simulink model "s_heli_2d_ff_lqr_i"  (Simulink 7.0)
settings: Solver=ode1  StartTime=0.0  StopTime=50  FixedStep=0.002  RelTol=1e-3
values from neighbouring files (symbols this model uses):
  g = 9.81    [setup_heli_2d_configuration.m]
  J_eq_p = J_m_p + J_body_p + J_p + J_y    (= 0.0384309870395)    [setup_heli_2d_configuration.m]
  J_eq_y = J_m_y + J_body_y + J_p + J_y + J_shaft    (= 0.0431517259335)    [setup_heli_2d_configuration.m]
  K_pp = K_f_p * r_p    (= 0.20413345)    [setup_heli_2d_configuration.m]
  K_py = K_t_y / R_m_y    (= 0.0068125)    [setup_heli_2d_configuration.m]
  K_yp = K_t_p / R_m_p    (= 0.0219277108434)    [setup_heli_2d_configuration.m]
  K_yy = K_f_y * r_y    (= 0.071988045)    [setup_heli_2d_configuration.m]
  l_cm = ( (m_motor_p + m_shield ) * r_p +  (m_motor_y + m_shield ) * r_y ) / ( m_props )    (= 0.185670125995)    [setup_heli_2d_configuration.m]
  m_heli = 1.3872    [setup_heli_2d_configuration.m]
  SAT_INT_ERR_PITCH = 8    [setup_lab_heli_2d.m]
  SAT_INT_ERR_YAW = 8    [setup_lab_heli_2d.m]
  theta_0 = -40.5*pi/180    (= -0.706858347058)    [setup_lab_heli_2d.m]
  Tr_p = 1    [setup_lab_heli_2d.m]
  Tr_y = 1    [setup_lab_heli_2d.m]
  VMAX_AMP_P = 24    [setup_lab_heli_2d.m]
  VMAX_AMP_Y = 15    [setup_lab_heli_2d.m]
undefined symbols (not defined in the file or in its folder): B_p, B_y, K, Ki
libraries: simulink x4, simulink_extras x4
settings Model: Creator=MLevis  LastModifiedBy=MLevis  ExtModeTrigDuration=5000
settings SolverCC: PositivePriorityOrder=on
settings DebuggingCC: SaveWithParameterizedLinksMsg=none
settings RTWCC: SystemTargetFile=quarc_windows.tlc  TemplateMakefile=quarc_default_tmf  Description=QUARC Win32 Target  ProcessScript=quarc_windows_make_rtw_hook
settings STFCustomTargetCC: TargetFcnLib=ansi_tfl_tmw.mat  TargetPreCompLibLocation=C:\DOCUME~1\ALLUSE~1\APPLIC~1\QUARC\lib\2007b\windows\release  GenFloatMathFcnCalls=ANSI_C  SystemTargetFile=quarc_windows.tlc
settings GRTTargetCC: TargetFcnLib=ansi_tfl_tmw.mat  TargetPreCompLibLocation=C:\DOCUME~1\ALLUSE~1\APPLIC~1\QUARC\lib\2007b\windows\release  CompOptLevelCompliant=off  MatFileLogging=off  ExtMode=on  ExtModeMexFile=quarc_comm

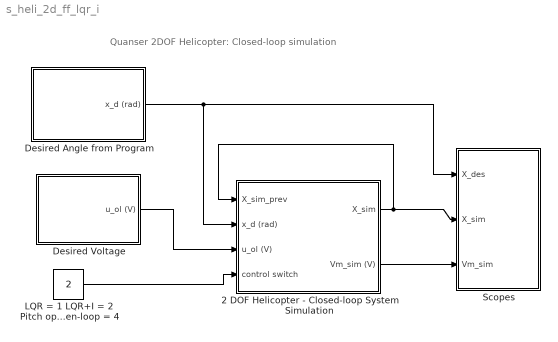
== system s_heli_2d_ff_lqr_i ==
  note: Quanser 2DOF Helicopter: Closed-loop simulation
  2 DOF Helicopter - Closed-loop System Simulation : Subsystem
  Desired Angle from Program : Subsystem
  Desired Voltage : Subsystem
  LQR = 1 LQR+I = 2 Pitch open-loop  = 3 Yaw open-loop = 4 : Constant  Value=2  OutDataType=sfix(16)  OutScaling=2^0
  Scopes : Subsystem
  wires:
  2 DOF Helicopter - Closed-loop System Simulation/1(X_sim) -> 2 DOF Helicopter - Closed-loop System Simulation/1(X_sim_prev), Scopes/2(X_sim)
  2 DOF Helicopter - Closed-loop System Simulation/2(Vm_sim (V)) -> Scopes/3(Vm_sim)
  Desired Angle from Program/1(x_d (rad)) -> Scopes/1(X_des), 2 DOF Helicopter - Closed-loop System Simulation/2(x_d (rad))
  LQR = 1 LQR+I = 2 Pitch open-loop  = 3 Yaw open-loop = 4/1 -> 2 DOF Helicopter - Closed-loop System Simulation/4(control switch)
  Desired Voltage/1(u_ol (V)) -> 2 DOF Helicopter - Closed-loop System Simulation/3(u_ol (V))

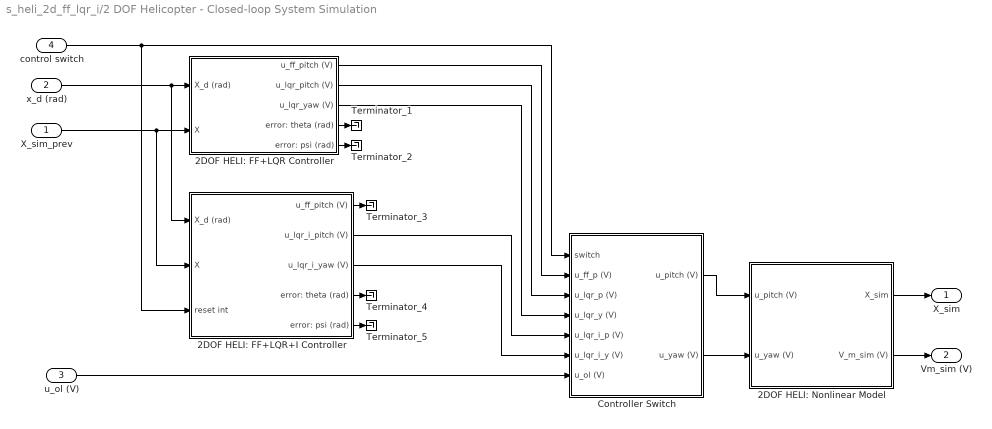
== system s_heli_2d_ff_lqr_i/2 DOF Helicopter - Closed-loop System Simulation ==
  X_sim_prev : Inport  OutDataType=sfix(16)  OutScaling=2^0
  x_d (rad) : Inport  Port=2  OutDataType=sfix(16)  OutScaling=2^0
  u_ol (V) : Inport  Port=3  OutDataType=sfix(16)  OutScaling=2^0
  control switch : Inport  Port=4  OutDataType=sfix(16)  OutScaling=2^0
  2DOF HELI: FF+LQR Controller : Subsystem
  2DOF HELI: FF+LQR+I Controller : Subsystem
  2DOF HELI: Nonlinear Model : Subsystem
  Controller Switch : Subsystem
  Terminator_{1..5} (5 alike) : Terminator
  X_sim : Outport  OutDataType=sfix(16)  OutScaling=2^0
  Vm_sim (V) : Outport  Port=2  OutDataType=sfix(16)  OutScaling=2^0
  wires:
  u_ol (V)/1 -> Controller Switch/7(u_ol (V))
  Controller Switch/2(u_yaw (V)) -> 2DOF HELI: Nonlinear Model/2(u_yaw (V))
  Controller Switch/1(u_pitch (V)) -> 2DOF HELI: Nonlinear Model/1(u_pitch (V))
  x_d (rad)/1 -> 2DOF HELI: FF+LQR+I Controller/1(X_d (rad)), 2DOF HELI: FF+LQR Controller/1(X_d (rad))
  X_sim_prev/1 -> 2DOF HELI: FF+LQR+I Controller/2(X), 2DOF HELI: FF+LQR Controller/2(X)
  2DOF HELI: FF+LQR+I Controller/3(u_lqr_i_yaw (V)) -> Controller Switch/6(u_lqr_i_y (V))
  2DOF HELI: FF+LQR Controller/2(u_lqr_pitch (V)) -> Controller Switch/3(u_lqr_p (V))
  2DOF HELI: FF+LQR Controller/1(u_ff_pitch (V)) -> Controller Switch/2(u_ff_p (V))
  2DOF HELI: FF+LQR Controller/3(u_lqr_yaw (V)) -> Controller Switch/4(u_lqr_y (V))
  2DOF HELI: FF+LQR+I Controller/2(u_lqr_i_pitch (V)) -> Controller Switch/5(u_lqr_i_p (V))
  control switch/1 -> Controller Switch/1(switch), 2DOF HELI: FF+LQR+I Controller/3(reset int)
  2DOF HELI: Nonlinear Model/2(V_m_sim (V)) -> Vm_sim (V)/1
  2DOF HELI: Nonlinear Model/1(X_sim) -> X_sim/1
  2DOF HELI: FF+LQR Controller/4(error: theta (rad)) -> Terminator_1/1
  2DOF HELI: FF+LQR Controller/5(error: psi (rad)) -> Terminator_2/1
  2DOF HELI: FF+LQR+I Controller/1(u_ff_pitch (V)) -> Terminator_3/1
  2DOF HELI: FF+LQR+I Controller/4(error: theta (rad)) -> Terminator_4/1
  2DOF HELI: FF+LQR+I Controller/5(error: psi (rad)) -> Terminator_5/1

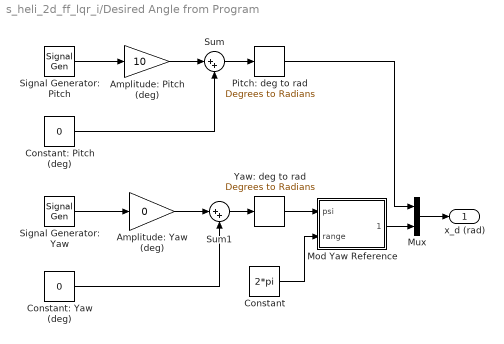
== system s_heli_2d_ff_lqr_i/Desired Angle from Program ==
  Amplitude: Pitch (deg) : Gain  Gain=10  ParameterDataType=sfix(16)  ParameterScaling=2^0  OutDataType=sfix(16)  OutScaling=2^0
  Amplitude: Yaw (deg) : Gain  Gain=0  ParameterDataType=sfix(16)  ParameterScaling=2^0  OutDataType=sfix(16)  OutScaling=2^0
  Constant : Constant  Value=2*pi  OutDataType=sfix(16)  OutScaling=2^0
  Constant: Pitch (deg) : Constant  Value=0  OutDataType=sfix(16)  OutScaling=2^0
  Constant: Yaw (deg) : Constant  Value=0  OutDataType=sfix(16)  OutScaling=2^0
  Mod Yaw Reference : Subsystem
  Mux : Mux  Inputs=2
  Pitch: deg to rad : simulink_extras/Transformations/Degrees to Radians  SystemSampleTime=-1
  Signal Generator: Pitch : SignalGenerator  WaveForm=square  Frequency=0.05
  Signal Generator: Yaw : SignalGenerator  WaveForm=square  Frequency=0.05
  Sum : Sum  Inputs=|++  OutDataType=sfix(16)  OutScaling=2^0
  Sum1 : Sum  Inputs=|++  OutDataType=sfix(16)  OutScaling=2^0
  Yaw: deg to rad : simulink_extras/Transformations/Degrees to Radians  SystemSampleTime=-1
  x_d (rad) : Outport  OutDataType=sfix(16)  OutScaling=2^0
  wires:
  Constant/1 -> Mod Yaw Reference/2(range)
  Yaw: deg to rad/1 -> Mod Yaw Reference/1(psi)
  Mod Yaw Reference/1(mod psi) -> Mux/2
  Pitch: deg to rad/1 -> Mux/1
  Sum/1 -> Pitch: deg to rad/1
  Signal Generator: Pitch/1 -> Amplitude: Pitch (deg)/1
  Amplitude: Pitch (deg)/1 -> Sum/1
  Constant: Pitch (deg)/1 -> Sum/2
  Sum1/1 -> Yaw: deg to rad/1
  Signal Generator: Yaw/1 -> Amplitude: Yaw (deg)/1
  Amplitude: Yaw (deg)/1 -> Sum1/1
  Constant: Yaw (deg)/1 -> Sum1/2
  Mux/1 -> x_d (rad)/1

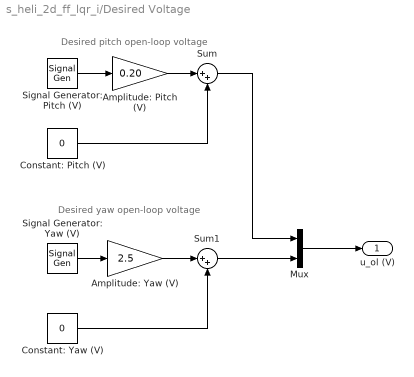
== system s_heli_2d_ff_lqr_i/Desired Voltage ==
  note: Desired pitch open-loop voltage
  note: Desired yaw open-loop voltage
  Amplitude: Pitch (V) : Gain  Gain=0.20  ParameterDataType=sfix(16)  ParameterScaling=2^0  OutDataType=sfix(16)  OutScaling=2^0
  Amplitude: Yaw (V) : Gain  Gain=2.5  ParameterDataType=sfix(16)  ParameterScaling=2^0  OutDataType=sfix(16)  OutScaling=2^0
  Constant: Pitch (V) : Constant  Value=0  OutDataType=sfix(16)  OutScaling=2^0
  Constant: Yaw (V) : Constant  Value=0  OutDataType=sfix(16)  OutScaling=2^0
  Mux : Mux  Inputs=2
  Signal Generator: Pitch (V) : SignalGenerator  WaveForm=square  Frequency=0.5
  Signal Generator: Yaw (V) : SignalGenerator  WaveForm=square  Frequency=0.01
  Sum : Sum  Inputs=|++  OutDataType=sfix(16)  OutScaling=2^0
  Sum1 : Sum  Inputs=|++  OutDataType=sfix(16)  OutScaling=2^0
  u_ol (V) : Outport  OutDataType=sfix(16)  OutScaling=2^0
  wires:
  Constant: Pitch (V)/1 -> Sum/2
  Amplitude: Pitch (V)/1 -> Sum/1
  Signal Generator: Pitch (V)/1 -> Amplitude: Pitch (V)/1
  Constant: Yaw (V)/1 -> Sum1/2
  Amplitude: Yaw (V)/1 -> Sum1/1
  Signal Generator: Yaw (V)/1 -> Amplitude: Yaw (V)/1
  Sum/1 -> Mux/1
  Sum1/1 -> Mux/2
  Mux/1 -> u_ol (V)/1

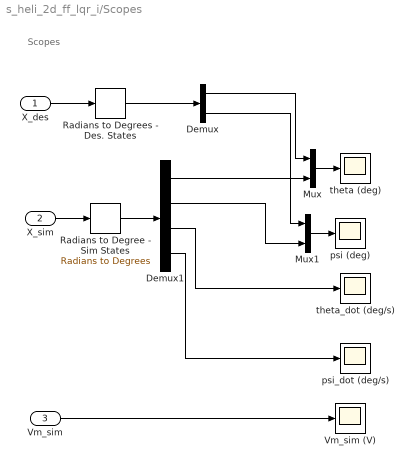
== system s_heli_2d_ff_lqr_i/Scopes ==
  note: Scopes
  X_des : Inport  OutDataType=sfix(16)  OutScaling=2^0
  X_sim : Inport  Port=2  OutDataType=sfix(16)  OutScaling=2^0
  Vm_sim : Inport  Port=3  OutDataType=sfix(16)  OutScaling=2^0
  Demux : Demux  Outputs=2
  Demux1 : Demux
  Mux : Mux  Inputs=2
  Mux1 : Mux  Inputs=2
  Radians to Degree - Sim States : simulink_extras/Transformations/Radians to Degrees  SystemSampleTime=-1
  Radians to Degrees - Des. States : simulink_extras/Transformations/Radians to Degrees  SystemSampleTime=-1
  Vm_sim (V) : Scope
      settings: TickLabels=on  TimeRange=50  YMin=-25  YMax=25  SaveName=ScopeData5  DataFormat=Array
  psi (deg) : Scope
      settings: TickLabels=on  TimeRange=50  YMin=-80  YMax=80  DataFormat=Array
  psi_dot (deg/s) : Scope
      settings: TickLabels=on  TimeRange=50  YMin=-300  YMax=300  SaveName=ScopeData3  DataFormat=Array
  theta (deg) : Scope
      settings: TickLabels=on  TimeRange=50  YMin=-15  YMax=15  DataFormat=Array
  theta_dot (deg/s) : Scope
      settings: TickLabels=on  TimeRange=50  YMin=-300  YMax=300  SaveName=ScopeData2  DataFormat=Array
  wires:
  Vm_sim/1 -> Vm_sim (V)/1
  Radians to Degrees - Des. States/1 -> Demux/1
  Demux1/2 -> Mux1/2
  Demux/2 -> Mux1/1
  Demux1/1 -> Mux/2
  Demux/1 -> Mux/1
  X_des/1 -> Radians to Degrees - Des. States/1
  X_sim/1 -> Radians to Degree - Sim States/1
  Radians to Degree - Sim States/1 -> Demux1/1
  Mux/1 -> theta (deg)/1
  Mux1/1 -> psi (deg)/1
  Demux1/3 -> theta_dot (deg/s)/1
  Demux1/4 -> psi_dot (deg/s)/1

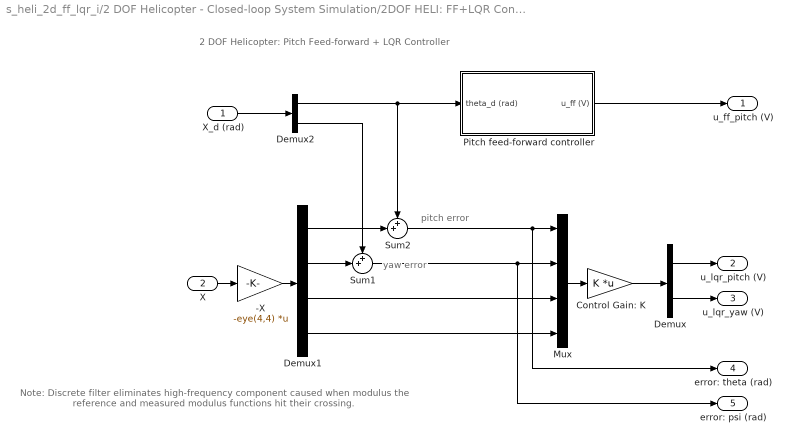
== system s_heli_2d_ff_lqr_i/2 DOF Helicopter - Closed-loop System Simulation/2DOF HELI: FF+LQR Controller ==
  note: Note: Discrete filter eliminates high-frequency
      | component caused when modulus the reference
      | and measured modulus functions hit their crossing.
  note: 2 DOF Helicopter:
      | Pitch Feed-forward + LQR Controller
  note: pitch error
  note: yaw error
  X_d (rad) : Inport  OutDataType=sfix(16)  OutScaling=2^0
  X : Inport  Port=2  OutDataType=sfix(16)  OutScaling=2^0
  -X : Gain  Gain=-eye(4,4)  Multiplication=Matrix(K*u)  ParameterDataType=sfix(16)  ParameterScaling=2^0  OutDataType=sfix(16)  OutScaling=2^0
  Control Gain: K : Gain  Gain=K  Multiplication=Matrix(K*u)  ParameterDataType=sfix(16)  ParameterScaling=2^0  OutDataType=sfix(16)  OutScaling=2^0
  Demux : Demux  Outputs=2
  Demux1 : Demux
  Demux2 : Demux  Outputs=2
  Mux : Mux
  Pitch feed-forward controller : Subsystem
  Sum1 : Sum  Inputs=++|  OutDataType=sfix(16)  OutScaling=2^0
  Sum2 : Sum  Inputs=++|  OutDataType=sfix(16)  OutScaling=2^0
  u_ff_pitch (V) : Outport  OutDataType=sfix(16)  OutScaling=2^0
  u_lqr_pitch (V) : Outport  Port=2  OutDataType=sfix(16)  OutScaling=2^0
  u_lqr_yaw (V) : Outport  Port=3  OutDataType=sfix(16)  OutScaling=2^0
  error: theta (rad) : Outport  Port=4  OutDataType=sfix(16)  OutScaling=2^0
  error: psi (rad) : Outport  Port=5  OutDataType=sfix(16)  OutScaling=2^0
  wires:
  Sum1/1 -> error: psi (rad)/1, Mux/2
  Demux2/1 -> Sum2/1, Pitch feed-forward controller/1(theta_d (rad))
  Demux2/2 -> Sum1/1
  Demux1/2 -> Sum1/2
  X_d (rad)/1 -> Demux2/1
  Demux1/4 -> Mux/4
  Demux1/3 -> Mux/3
  Mux/1 -> Control Gain: K/1
  Control Gain: K/1 -> Demux/1
  -X/1 -> Demux1/1
  X/1 -> -X/1
  Demux1/1 -> Sum2/2
  Sum2/1 -> error: theta (rad)/1, Mux/1
  Demux/2 -> u_lqr_yaw (V)/1
  Demux/1 -> u_lqr_pitch (V)/1
  Pitch feed-forward controller/1(u_ff (V)) -> u_ff_pitch (V)/1

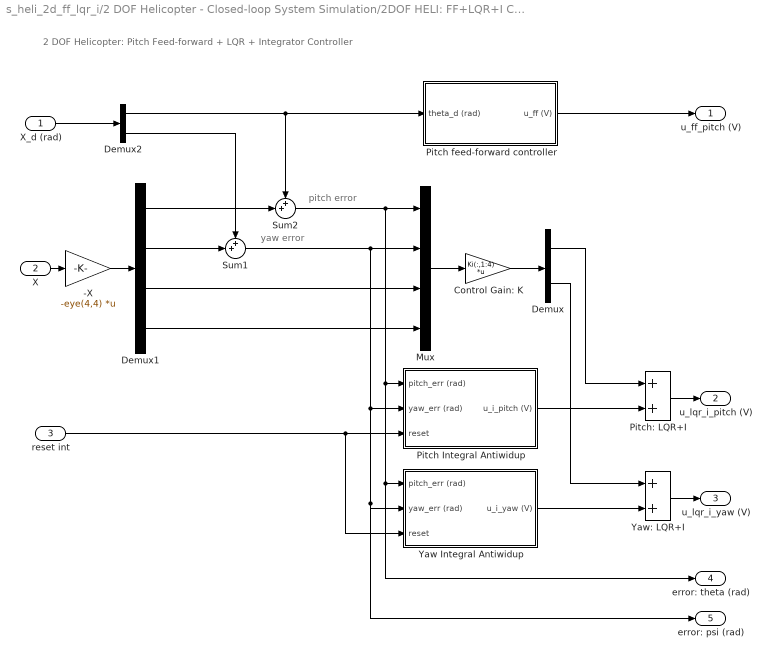
== system s_heli_2d_ff_lqr_i/2 DOF Helicopter - Closed-loop System Simulation/2DOF HELI: FF+LQR+I Controller ==
  note: yaw error
  note: pitch error
  note: 2 DOF Helicopter:
      | Pitch Feed-forward + LQR + Integrator Controller
  X_d (rad) : Inport  OutDataType=sfix(16)  OutScaling=2^0
  X : Inport  Port=2  OutDataType=sfix(16)  OutScaling=2^0
  reset int : Inport  Port=3  OutDataType=sfix(16)  OutScaling=2^0
  -X : Gain  Gain=-eye(4,4)  Multiplication=Matrix(K*u)  ParameterDataType=sfix(16)  ParameterScaling=2^0  OutDataType=sfix(16)  OutScaling=2^0
  Control Gain: K : Gain  Gain=Ki(:,1:4)  Multiplication=Matrix(K*u)  ParameterDataType=sfix(16)  ParameterScaling=2^0  OutDataType=sfix(16)  OutScaling=2^0
  Demux : Demux  Outputs=2
  Demux1 : Demux
  Demux2 : Demux  Outputs=2
  Mux : Mux
  Pitch Integral Antiwidup : Subsystem
  Pitch feed-forward controller : Subsystem
  Pitch: LQR+I : Sum  OutDataType=sfix(16)  OutScaling=2^-10
  Sum1 : Sum  Inputs=++|  OutDataType=sfix(16)  OutScaling=2^0
  Sum2 : Sum  Inputs=++|  OutDataType=sfix(16)  OutScaling=2^0
  Yaw Integral Antiwidup : Subsystem
  Yaw: LQR+I : Sum  OutDataType=sfix(16)  OutScaling=2^-10
  u_ff_pitch (V) : Outport  OutDataType=sfix(16)  OutScaling=2^0
  u_lqr_i_pitch (V) : Outport  Port=2  OutDataType=sfix(16)  OutScaling=2^0
  u_lqr_i_yaw (V) : Outport  Port=3  OutDataType=sfix(16)  OutScaling=2^0
  error: theta (rad) : Outport  Port=4  OutDataType=sfix(16)  OutScaling=2^0
  error: psi (rad) : Outport  Port=5  OutDataType=sfix(16)  OutScaling=2^0
  wires:
  reset int/1 -> Pitch Integral Antiwidup/3(reset), Yaw Integral Antiwidup/3(reset)
  Demux1/2 -> Sum1/2
  Demux2/2 -> Sum1/1
  Demux2/1 -> Sum2/1, Pitch feed-forward controller/1(theta_d (rad))
  X_d (rad)/1 -> Demux2/1
  Yaw Integral Antiwidup/1(u_i_yaw (V)) -> Yaw: LQR+I/2
  Demux/2 -> Yaw: LQR+I/1
  Yaw: LQR+I/1 -> u_lqr_i_yaw (V)/1
  Pitch: LQR+I/1 -> u_lqr_i_pitch (V)/1
  Demux/1 -> Pitch: LQR+I/1
  Pitch Integral Antiwidup/1(u_i_pitch (V)) -> Pitch: LQR+I/2
  Pitch feed-forward controller/1(u_ff (V)) -> u_ff_pitch (V)/1
  Sum2/1 -> Mux/1, Yaw Integral Antiwidup/1(pitch_err (rad)), error: theta (rad)/1, Pitch Integral Antiwidup/1(pitch_err (rad))
  Demux1/1 -> Sum2/2
  X/1 -> -X/1
  Sum1/1 -> Yaw Integral Antiwidup/2(yaw_err (rad)), error: psi (rad)/1, Pitch Integral Antiwidup/2(yaw_err (rad)), Mux/2
  -X/1 -> Demux1/1
  Control Gain: K/1 -> Demux/1
  Mux/1 -> Control Gain: K/1
  Demux1/3 -> Mux/3
  Demux1/4 -> Mux/4

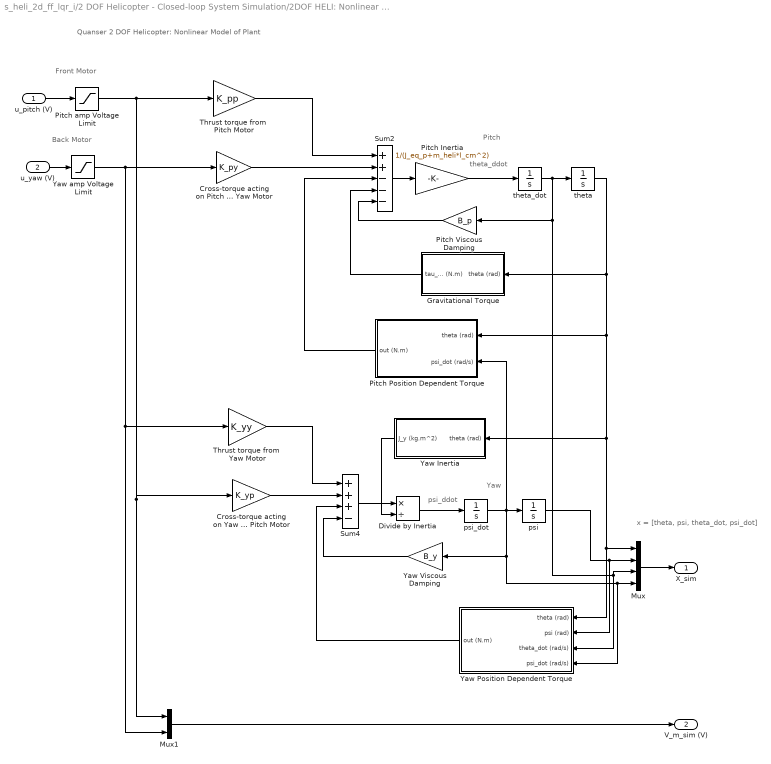
== system s_heli_2d_ff_lqr_i/2 DOF Helicopter - Closed-loop System Simulation/2DOF HELI: Nonlinear Model ==
  note: Yaw
  note: Pitch
  note: psi_ddot
  note: theta_ddot
  note: Quanser 2 DOF Helicopter: Nonlinear Model of Plant
  note: x = [theta, psi, theta_dot, psi_dot]
  note: Front Motor
  note: Back Motor
  u_pitch (V) : Inport  OutDataType=sfix(16)  OutScaling=2^0
  u_yaw (V) : Inport  Port=2  OutDataType=sfix(16)  OutScaling=2^0
  Cross-torque acting on Pitch  from Yaw Motor : Gain  Gain=K_py  ParameterDataType=sfix(16)  ParameterScaling=2^0  OutDataType=sfix(16)  OutScaling=2^0
  Cross-torque acting on Yaw  from Pitch Motor : Gain  Gain=K_yp  ParameterDataType=sfix(16)  ParameterScaling=2^0  OutDataType=sfix(16)  OutScaling=2^0
  Divide by Inertia : Product  Inputs=*/  OutDataType=sfix(16)  OutScaling=2^-10
  Gravitational Torque : Subsystem  Orientation=left
  Mux : Mux
  Mux1 : Mux  Inputs=2
  Pitch Inertia : Gain  Gain=1/(J_eq_p+m_heli*l_cm^2)  ParameterDataType=sfix(16)  ParameterScaling=2^0  OutDataType=sfix(16)  OutScaling=2^0
  Pitch Position Dependent Torque : Subsystem  Orientation=left
  Pitch Viscous Damping : Gain  Orientation=left  Gain=B_p  ParameterDataType=sfix(16)  ParameterScaling=2^0  OutDataType=sfix(16)  OutScaling=2^0
  Pitch amp Voltage Limit : Saturate  UpperLimit=VMAX_AMP_P  LowerLimit=- VMAX_AMP_P
  Sum2 : Sum  Inputs=++---  OutDataType=sfix(16)  OutScaling=2^0
  Sum4 : Sum  Inputs=+++-  OutDataType=sfix(16)  OutScaling=2^0
  Thrust torque from  Pitch Motor : Gain  Gain=K_pp  ParameterDataType=sfix(16)  ParameterScaling=2^0  OutDataType=sfix(16)  OutScaling=2^0
  Thrust torque from  Yaw Motor : Gain  Gain=K_yy  ParameterDataType=sfix(16)  ParameterScaling=2^0  OutDataType=sfix(16)  OutScaling=2^0
  Yaw Inertia : Subsystem  Orientation=left
  Yaw Position Dependent Torque : Subsystem  Orientation=left
  Yaw Viscous Damping : Gain  Orientation=left  Gain=B_y  ParameterDataType=sfix(16)  ParameterScaling=2^0  OutDataType=sfix(16)  OutScaling=2^0
  Yaw amp Voltage Limit : Saturate  UpperLimit=VMAX_AMP_Y  LowerLimit=- VMAX_AMP_Y
  psi : Integrator
  psi_dot : Integrator
  theta : Integrator  InitialCondition=theta_0  LimitOutput=on  UpperSaturationLimit=40.5*pi/180  LowerSaturationLimit=-40.5*pi/180
  theta_dot : Integrator
  X_sim : Outport  OutDataType=sfix(16)  OutScaling=2^0
  V_m_sim (V) : Outport  Port=2  OutDataType=sfix(16)  OutScaling=2^0
  wires:
  u_yaw (V)/1 -> Yaw amp Voltage Limit/1
  u_pitch (V)/1 -> Pitch amp Voltage Limit/1
  psi_dot/1 -> psi/1, Pitch Position Dependent Torque/2(psi_dot (rad/s)), Mux/4, Yaw Position Dependent Torque/4(psi_dot (rad/s)), Yaw Viscous Damping/1
  Cross-torque acting on Yaw  from Pitch Motor/1 -> Sum4/2
  Thrust torque from  Yaw Motor/1 -> Sum4/1
  theta_dot/1 -> theta/1, Mux/3, Yaw Position Dependent Torque/3(theta_dot (rad/s)), Pitch Viscous Damping/1
  Pitch Inertia/1 -> theta_dot/1
  Sum2/1 -> Pitch Inertia/1
  theta/1 -> Yaw Inertia/1(theta (rad)), Mux/1, Yaw Position Dependent Torque/1(theta (rad)), Pitch Position Dependent Torque/1(theta (rad)), Gravitational Torque/1(theta (rad))
  Mux/1 -> X_sim/1
  Pitch amp Voltage Limit/1 -> Thrust torque from  Pitch Motor/1, Mux1/1, Cross-torque acting on Yaw  from Pitch Motor/1
  Yaw amp Voltage Limit/1 -> Cross-torque acting on Pitch  from Yaw Motor/1, Mux1/2, Thrust torque from  Yaw Motor/1
  Mux1/1 -> V_m_sim (V)/1
  psi/1 -> Mux/2, Yaw Position Dependent Torque/2(psi (rad))
  Yaw Viscous Damping/1 -> Sum4/4
  Yaw Position Dependent Torque/1(out (N.m)) -> Sum4/3
  Sum4/1 -> Divide by Inertia/1
  Divide by Inertia/1 -> psi_dot/1
  Yaw Inertia/1(J_y (kg.m^2)) -> Divide by Inertia/2
  Thrust torque from  Pitch Motor/1 -> Sum2/1
  Cross-torque acting on Pitch  from Yaw Motor/1 -> Sum2/2
  Pitch Viscous Damping/1 -> Sum2/5
  Gravitational Torque/1(tau_g (N.m)) -> Sum2/4
  Pitch Position Dependent Torque/1(out (N.m)) -> Sum2/3

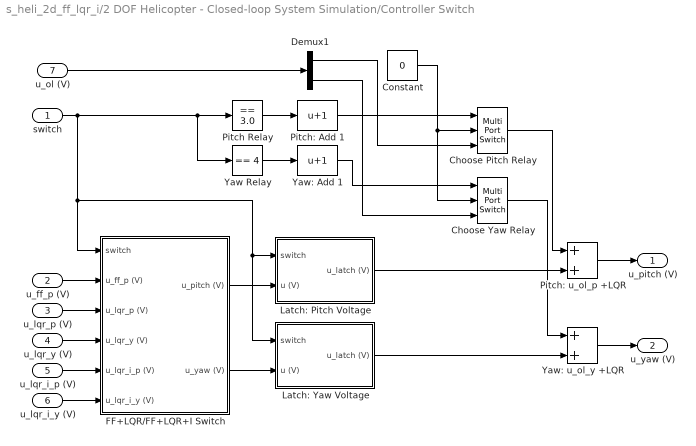
== system s_heli_2d_ff_lqr_i/2 DOF Helicopter - Closed-loop System Simulation/Controller Switch ==
  switch : Inport  OutDataType=sfix(16)  OutScaling=2^0
  u_ff_p (V) : Inport  Port=2  OutDataType=sfix(16)  OutScaling=2^0
  u_lqr_p (V) : Inport  Port=3  OutDataType=sfix(16)  OutScaling=2^0
  u_lqr_y (V) : Inport  Port=4  OutDataType=sfix(16)  OutScaling=2^0
  u_lqr_i_p (V) : Inport  Port=5  OutDataType=sfix(16)  OutScaling=2^0
  u_lqr_i_y (V) : Inport  Port=6  OutDataType=sfix(16)  OutScaling=2^0
  u_ol (V) : Inport  Port=7  OutDataType=sfix(16)  OutScaling=2^0
  Choose Pitch Relay : MultiPortSwitch  Inputs=2
  Choose Yaw Relay : MultiPortSwitch  Inputs=2
  Constant : Constant  Value=0  OutDataType=sfix(16)  OutScaling=2^0
  Demux1 : Demux  Outputs=2
  FF+LQR/FF+LQR+I Switch : Subsystem
  Latch: Pitch Voltage : Subsystem
  Latch: Yaw Voltage : Subsystem
  Pitch Relay : simulink/Logic and Bit Operations/Compare To Constant  SystemSampleTime=-1  relop===  const=3.0  LogicOutDataTypeMode=uint8  ZeroCross=off
  Pitch: u_ol_p +LQR : Sum  OutDataType=sfix(16)  OutScaling=2^-10
  Pitch: Add 1 : Bias  Bias=1
  Yaw Relay : simulink/Logic and Bit Operations/Compare To Constant  SystemSampleTime=-1  relop===  const=4  LogicOutDataTypeMode=uint8  ZeroCross=off
  Yaw: u_ol_y +LQR : Sum  OutDataType=sfix(16)  OutScaling=2^-10
  Yaw: Add 1 : Bias  Bias=1
  u_pitch (V) : Outport  OutDataType=sfix(16)  OutScaling=2^0
  u_yaw (V) : Outport  Port=2  OutDataType=sfix(16)  OutScaling=2^0
  wires:
  Choose Pitch Relay/1 -> Pitch: u_ol_p +LQR/1
  Choose Yaw Relay/1 -> Yaw: u_ol_y +LQR/1
  Demux1/2 -> Choose Yaw Relay/3
  Demux1/1 -> Choose Pitch Relay/3
  Constant/1 -> Choose Yaw Relay/2, Choose Pitch Relay/2
  Yaw: Add 1/1 -> Choose Yaw Relay/1
  Yaw Relay/1 -> Yaw: Add 1/1
  u_ol (V)/1 -> Demux1/1
  Pitch: Add 1/1 -> Choose Pitch Relay/1
  Pitch Relay/1 -> Pitch: Add 1/1
  Yaw: u_ol_y +LQR/1 -> u_yaw (V)/1
  Pitch: u_ol_p +LQR/1 -> u_pitch (V)/1
  switch/1 -> Yaw Relay/1, Pitch Relay/1, Latch: Yaw Voltage/1(switch), Latch: Pitch Voltage/1(switch), FF+LQR/FF+LQR+I Switch/1(switch)
  Latch: Yaw Voltage/1(u_latch (V)) -> Yaw: u_ol_y +LQR/2
  Latch: Pitch Voltage/1(u_latch (V)) -> Pitch: u_ol_p +LQR/2
  u_lqr_i_y (V)/1 -> FF+LQR/FF+LQR+I Switch/6(u_lqr_i_y (V))
  u_lqr_i_p (V)/1 -> FF+LQR/FF+LQR+I Switch/5(u_lqr_i_p (V))
  u_lqr_y (V)/1 -> FF+LQR/FF+LQR+I Switch/4(u_lqr_y (V))
  u_lqr_p (V)/1 -> FF+LQR/FF+LQR+I Switch/3(u_lqr_p (V))
  u_ff_p (V)/1 -> FF+LQR/FF+LQR+I Switch/2(u_ff_p (V))
  FF+LQR/FF+LQR+I Switch/2(u_yaw (V)) -> Latch: Yaw Voltage/2(u (V))
  FF+LQR/FF+LQR+I Switch/1(u_pitch (V)) -> Latch: Pitch Voltage/2(u (V))

== system s_heli_2d_ff_lqr_i/Desired Angle from Program/Mod Yaw Reference ==
  psi : Inport  OutDataType=sfix(16)  OutScaling=2^0
  range : Inport  Port=2  OutDataType=sfix(16)  OutScaling=2^0
  Math Function : Math  Operator=mod  OutDataType=sfix(16)  OutScaling=2^0  SaturateOnIntegerOverflow=on
  Product : Product  OutDataType=sfix(16)  OutScaling=2^0  RndMeth=Zero
  Sign : Signum
  mod psi : Outport  OutDataType=sfix(16)  OutScaling=2^0
  wires:
  range/1 -> Product/2
  Math Function/1 -> mod psi/1
  psi/1 -> Sign/1, Math Function/1
  Sign/1 -> Product/1
  Product/1 -> Math Function/2

== system s_heli_2d_ff_lqr_i/2 DOF Helicopter - Closed-loop System Simulation/2DOF HELI: FF+LQR Controller/Pitch feed-forward controller ==
  note: Desired pitch angle
  theta_d (rad) : Inport  OutDataType=sfix(16)  OutScaling=2^0
  Feed-forward Pitch Gain : Gain  Gain=l_cm*m_heli*g / K_pp  ParameterDataType=sfix(16)  ParameterScaling=2^0  OutDataType=sfix(16)  OutScaling=2^0
  Trigonometric Function : Trigonometry  Operator=cos  OutputSignalType=real
  u_ff (V) : Outport  OutDataType=sfix(16)  OutScaling=2^0
  wires:
  theta_d (rad)/1 -> Trigonometric Function/1
  Feed-forward Pitch Gain/1 -> u_ff (V)/1
  Trigonometric Function/1 -> Feed-forward Pitch Gain/1

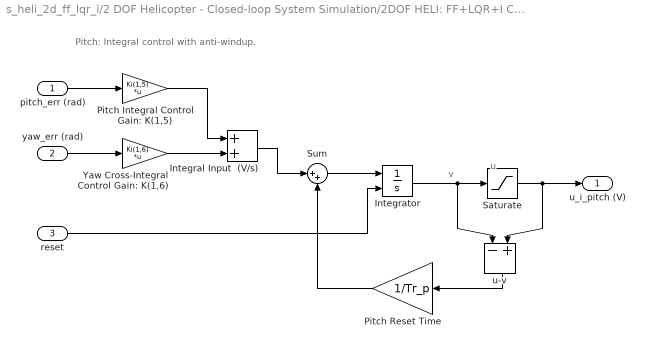
== system s_heli_2d_ff_lqr_i/2 DOF Helicopter - Closed-loop System Simulation/2DOF HELI: FF+LQR+I Controller/Pitch Integral Antiwidup ==
  note: Pitch: Integral control with anti-windup.
  note: v
  note: u
  pitch_err (rad) : Inport  OutDataType=sfix(16)  OutScaling=2^0
  yaw_err (rad) : Inport  Port=2  OutDataType=sfix(16)  OutScaling=2^0
  reset : Inport  Port=3  OutDataType=sfix(16)  OutScaling=2^0
  Integral Input  (V/s) : Sum  OutDataType=sfix(16)  OutScaling=2^-10
  Integrator : Integrator  ExternalReset=rising
  Pitch Integral Control Gain: K(1,5) : Gain  Gain=Ki(1,5)  Multiplication=Matrix(K*u)  ParameterDataType=sfix(16)  ParameterScaling=2^0  OutDataType=sfix(16)  OutScaling=2^0
  Pitch Reset Time : Gain  Orientation=left  Gain=1/Tr_p  ParameterDataType=sfix(16)  ParameterScaling=2^0  OutDataType=sfix(16)  OutScaling=2^0
  Saturate : Saturate  UpperLimit=SAT_INT_ERR_PITCH  LowerLimit=-SAT_INT_ERR_PITCH
  Sum : Sum  Inputs=|++  OutDataType=sfix(16)  OutScaling=2^0
  Yaw Cross-Integral Control Gain: K(1,6) : Gain  Gain=Ki(1,6)  Multiplication=Matrix(K*u)  ParameterDataType=sfix(16)  ParameterScaling=2^0  OutDataType=sfix(16)  OutScaling=2^0
  u-v : Sum  Orientation=down  Inputs=-+  OutDataType=sfix(16)  OutScaling=2^-10
  u_i_pitch (V) : Outport  OutDataType=sfix(16)  OutScaling=2^0
  wires:
  Integral Input  (V/s)/1 -> Sum/1
  Yaw Cross-Integral Control Gain: K(1,6)/1 -> Integral Input  (V/s)/2
  Pitch Integral Control Gain: K(1,5)/1 -> Integral Input  (V/s)/1
  yaw_err (rad)/1 -> Yaw Cross-Integral Control Gain: K(1,6)/1
  reset/1 -> Integrator/2
  Pitch Reset Time/1 -> Sum/2
  Sum/1 -> Integrator/1
  u-v/1 -> Pitch Reset Time/1
  Saturate/1 -> u-v/2, u_i_pitch (V)/1
  Integrator/1 -> Saturate/1, u-v/1
  pitch_err (rad)/1 -> Pitch Integral Control Gain: K(1,5)/1

== system s_heli_2d_ff_lqr_i/2 DOF Helicopter - Closed-loop System Simulation/2DOF HELI: FF+LQR+I Controller/Pitch feed-forward controller ==
  note: Desired pitch angle
  theta_d (rad) : Inport  OutDataType=sfix(16)  OutScaling=2^0
  Feed-forward Pitch Gain : Gain  Gain=l_cm*m_heli*g / K_pp  ParameterDataType=sfix(16)  ParameterScaling=2^0  OutDataType=sfix(16)  OutScaling=2^0
  Trigonometric Function : Trigonometry  Operator=cos  OutputSignalType=real
  u_ff (V) : Outport  OutDataType=sfix(16)  OutScaling=2^0
  wires:
  theta_d (rad)/1 -> Trigonometric Function/1
  Feed-forward Pitch Gain/1 -> u_ff (V)/1
  Trigonometric Function/1 -> Feed-forward Pitch Gain/1

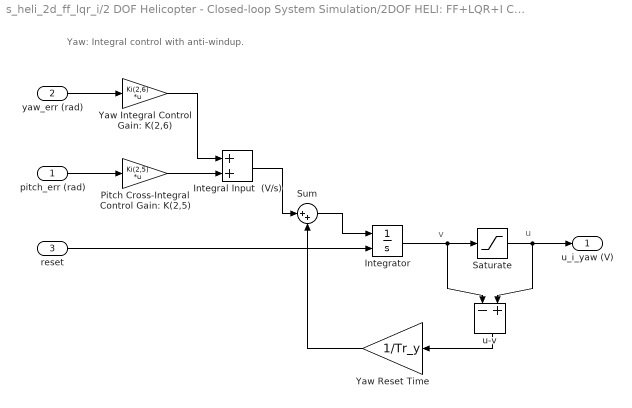
== system s_heli_2d_ff_lqr_i/2 DOF Helicopter - Closed-loop System Simulation/2DOF HELI: FF+LQR+I Controller/Yaw Integral Antiwidup ==
  note: Yaw: Integral control with anti-windup.
  note: u
  note: v
  pitch_err (rad) : Inport  OutDataType=sfix(16)  OutScaling=2^0
  yaw_err (rad) : Inport  Port=2  OutDataType=sfix(16)  OutScaling=2^0
  reset : Inport  Port=3  OutDataType=sfix(16)  OutScaling=2^0
  Integral Input  (V/s) : Sum  OutDataType=sfix(16)  OutScaling=2^-10
  Integrator : Integrator  ExternalReset=rising
  Pitch Cross-Integral Control Gain: K(2,5) : Gain  Gain=Ki(2,5)  Multiplication=Matrix(K*u)  ParameterDataType=sfix(16)  ParameterScaling=2^0  OutDataType=sfix(16)  OutScaling=2^0
  Saturate : Saturate  UpperLimit=SAT_INT_ERR_YAW  LowerLimit=-SAT_INT_ERR_YAW
  Sum : Sum  Inputs=|++  OutDataType=sfix(16)  OutScaling=2^0
  Yaw Integral Control Gain: K(2,6) : Gain  Gain=Ki(2,6)  Multiplication=Matrix(K*u)  ParameterDataType=sfix(16)  ParameterScaling=2^0  OutDataType=sfix(16)  OutScaling=2^0
  Yaw Reset Time : Gain  Orientation=left  Gain=1/Tr_y  ParameterDataType=sfix(16)  ParameterScaling=2^0  OutDataType=sfix(16)  OutScaling=2^0
  u-v : Sum  Orientation=down  Inputs=-+  OutDataType=sfix(16)  OutScaling=2^-10
  u_i_yaw (V) : Outport  OutDataType=sfix(16)  OutScaling=2^0
  wires:
  Integral Input  (V/s)/1 -> Sum/1
  Pitch Cross-Integral Control Gain: K(2,5)/1 -> Integral Input  (V/s)/2
  Yaw Integral Control Gain: K(2,6)/1 -> Integral Input  (V/s)/1
  pitch_err (rad)/1 -> Pitch Cross-Integral Control Gain: K(2,5)/1
  reset/1 -> Integrator/2
  yaw_err (rad)/1 -> Yaw Integral Control Gain: K(2,6)/1
  Integrator/1 -> u-v/1, Saturate/1
  Saturate/1 -> u_i_yaw (V)/1, u-v/2
  u-v/1 -> Yaw Reset Time/1
  Sum/1 -> Integrator/1
  Yaw Reset Time/1 -> Sum/2

== system s_heli_2d_ff_lqr_i/2 DOF Helicopter - Closed-loop System Simulation/2DOF HELI: Nonlinear Model/Gravitational Torque ==
  theta (rad) : Inport  OutDataType=sfix(16)  OutScaling=2^0
  Trigonometric Function : Trigonometry  Operator=cos  OutputSignalType=real
  m*g*lcm : Gain  Gain=m_heli*g*l_cm  ParameterDataType=sfix(16)  ParameterScaling=2^0  OutDataType=sfix(16)  OutScaling=2^0
  tau_g (N.m) : Outport  OutDataType=sfix(16)  OutScaling=2^0
  wires:
  Trigonometric Function/1 -> m*g*lcm/1
  theta (rad)/1 -> Trigonometric Function/1
  m*g*lcm/1 -> tau_g (N.m)/1

== system s_heli_2d_ff_lqr_i/2 DOF Helicopter - Closed-loop System Simulation/2DOF HELI: Nonlinear Model/Pitch Position Dependent Torque ==
  theta (rad) : Inport  OutDataType=sfix(16)  OutScaling=2^0
  psi_dot (rad/s) : Inport  Port=2  OutDataType=sfix(16)  OutScaling=2^0
  Product : Product  Inputs=4  OutDataType=sfix(16)  OutScaling=2^0  RndMeth=Zero
  cos(theta) : Trigonometry  Operator=cos  OutputSignalType=real
  m*lcm^2 : Gain  Gain=m_heli*l_cm^2  ParameterDataType=sfix(16)  ParameterScaling=2^0  OutDataType=sfix(16)  OutScaling=2^0
  sin(theta) : Trigonometry  OutputSignalType=real
  out (N.m) : Outport  OutDataType=sfix(16)  OutScaling=2^0
  wires:
  m*lcm^2/1 -> out (N.m)/1
  cos(theta)/1 -> Product/2
  sin(theta)/1 -> Product/1
  Product/1 -> m*lcm^2/1
  theta (rad)/1 -> sin(theta)/1, cos(theta)/1
  psi_dot (rad/s)/1 -> Product/3, Product/4

== system s_heli_2d_ff_lqr_i/2 DOF Helicopter - Closed-loop System Simulation/2DOF HELI: Nonlinear Model/Yaw Inertia ==
  theta (rad) : Inport  OutDataType=sfix(16)  OutScaling=2^0
  Sum3 : Sum  OutDataType=sfix(16)  OutScaling=2^0
  Yaw Inertia : Constant  Value=J_eq_y  OutDataType=sfix(16)  OutScaling=2^0
  cos(theta) : Trigonometry  Operator=cos  OutputSignalType=real
  cos(theta)^2 : Product  OutDataType=sfix(16)  OutScaling=2^0  RndMeth=Zero
  m_heli*l_cm^2 : Gain  Gain=m_heli*l_cm^2  ParameterDataType=sfix(16)  ParameterScaling=2^0  OutDataType=sfix(16)  OutScaling=2^0
  J_y (kg.m^2) : Outport  OutDataType=sfix(16)  OutScaling=2^0
  wires:
  cos(theta)^2/1 -> m_heli*l_cm^2/1
  Yaw Inertia/1 -> Sum3/1
  m_heli*l_cm^2/1 -> Sum3/2
  theta (rad)/1 -> cos(theta)/1
  Sum3/1 -> J_y (kg.m^2)/1
  cos(theta)/1 -> cos(theta)^2/1, cos(theta)^2/2

== system s_heli_2d_ff_lqr_i/2 DOF Helicopter - Closed-loop System Simulation/2DOF HELI: Nonlinear Model/Yaw Position Dependent Torque ==
  theta (rad) : Inport  OutDataType=sfix(16)  OutScaling=2^0
  psi (rad) : Inport  Port=2  OutDataType=sfix(16)  OutScaling=2^0
  theta_dot (rad/s) : Inport  Port=3  OutDataType=sfix(16)  OutScaling=2^0
  psi_dot (rad/s) : Inport  Port=4  OutDataType=sfix(16)  OutScaling=2^0
  2*m*lcm^2 : Gain  Gain=2*m_heli*l_cm^2  ParameterDataType=sfix(16)  ParameterScaling=2^0  OutDataType=sfix(16)  OutScaling=2^0
  Product : Product  Inputs=4  OutDataType=sfix(16)  OutScaling=2^0  RndMeth=Zero
  cos(theta) : Trigonometry  Operator=cos  OutputSignalType=real
  sin(psi) : Trigonometry  OutputSignalType=real
  out (N.m) : Outport  OutDataType=sfix(16)  OutScaling=2^0
  wires:
  psi (rad)/1 -> sin(psi)/1
  theta (rad)/1 -> cos(theta)/1
  Product/1 -> 2*m*lcm^2/1
  cos(theta)/1 -> Product/1
  sin(psi)/1 -> Product/2
  theta_dot (rad/s)/1 -> Product/3
  psi_dot (rad/s)/1 -> Product/4
  2*m*lcm^2/1 -> out (N.m)/1

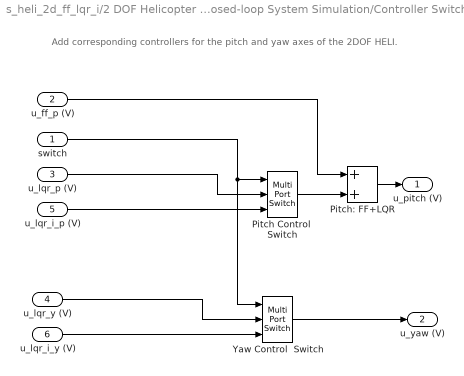
== system s_heli_2d_ff_lqr_i/2 DOF Helicopter - Closed-loop System Simulation/Controller Switch/FF+LQR/FF+LQR+I Switch ==
  note: Add corresponding controllers for the pitch and yaw axes of the 2DOF HELI.
  switch : Inport  OutDataType=sfix(16)  OutScaling=2^0
  u_ff_p (V) : Inport  Port=2  OutDataType=sfix(16)  OutScaling=2^0
  u_lqr_p (V) : Inport  Port=3  OutDataType=sfix(16)  OutScaling=2^0
  u_lqr_y (V) : Inport  Port=4  OutDataType=sfix(16)  OutScaling=2^0
  u_lqr_i_p (V) : Inport  Port=5  OutDataType=sfix(16)  OutScaling=2^0
  u_lqr_i_y (V) : Inport  Port=6  OutDataType=sfix(16)  OutScaling=2^0
  Pitch Control  Switch : MultiPortSwitch  Inputs=2
  Pitch: FF+LQR : Sum  OutDataType=sfix(16)  OutScaling=2^-10
  Yaw Control  Switch : MultiPortSwitch  Inputs=2
  u_pitch (V) : Outport  OutDataType=sfix(16)  OutScaling=2^0
  u_yaw (V) : Outport  Port=2  OutDataType=sfix(16)  OutScaling=2^0
  wires:
  switch/1 -> Yaw Control  Switch/1, Pitch Control  Switch/1
  u_lqr_i_y (V)/1 -> Yaw Control  Switch/3
  u_lqr_i_p (V)/1 -> Pitch Control  Switch/3
  Yaw Control  Switch/1 -> u_yaw (V)/1
  u_lqr_y (V)/1 -> Yaw Control  Switch/2
  u_lqr_p (V)/1 -> Pitch Control  Switch/2
  Pitch: FF+LQR/1 -> u_pitch (V)/1
  u_ff_p (V)/1 -> Pitch: FF+LQR/1
  Pitch Control  Switch/1 -> Pitch: FF+LQR/2

== system s_heli_2d_ff_lqr_i/2 DOF Helicopter - Closed-loop System Simulation/Controller Switch/Latch: Pitch Voltage ==
  switch : Inport  OutDataType=sfix(16)  OutScaling=2^0
  u (V) : Inport  Port=2  OutDataType=sfix(16)  OutScaling=2^0
  Add : Sum  OutDataType=sfix(16)  OutScaling=2^-10
  Compare To Constant : simulink/Logic and Bit Operations/Compare To Constant  SystemSampleTime=-1  relop=>=  const=3.0  LogicOutDataTypeMode=uint8  ZeroCross=off
  Constant : Constant  OutDataType=sfix(16)  OutScaling=2^0
  Memory : Memory  Orientation=left
  Switch : MultiPortSwitch  Inputs=2
  u_latch (V) : Outport  OutDataType=sfix(16)  OutScaling=2^0
  wires:
  Constant/1 -> Add/2
  Compare To Constant/1 -> Add/1
  switch/1 -> Compare To Constant/1
  u (V)/1 -> Switch/2
  Add/1 -> Switch/1
  Memory/1 -> Switch/3
  Switch/1 -> u_latch (V)/1, Memory/1

== system s_heli_2d_ff_lqr_i/2 DOF Helicopter - Closed-loop System Simulation/Controller Switch/Latch: Yaw Voltage ==
  switch : Inport  OutDataType=sfix(16)  OutScaling=2^0
  u (V) : Inport  Port=2  OutDataType=sfix(16)  OutScaling=2^0
  Add : Sum  OutDataType=sfix(16)  OutScaling=2^-10
  Compare To Constant : simulink/Logic and Bit Operations/Compare To Constant  SystemSampleTime=-1  relop=>=  const=3.0  LogicOutDataTypeMode=uint8  ZeroCross=off
  Constant : Constant  OutDataType=sfix(16)  OutScaling=2^0
  Memory : Memory  Orientation=left
  Switch : MultiPortSwitch  Inputs=2
  u_latch (V) : Outport  OutDataType=sfix(16)  OutScaling=2^0
  wires:
  Switch/1 -> Memory/1, u_latch (V)/1
  Memory/1 -> Switch/3
  Add/1 -> Switch/1
  u (V)/1 -> Switch/2
  switch/1 -> Compare To Constant/1
  Compare To Constant/1 -> Add/1
  Constant/1 -> Add/2
